simulink model "p1"  (R2020a)
settings: Solver=VariableStepAuto  StartTime=0.0  StopTime=10.0  RelTol=1e-3
settings Model: Creator=007  LastModifiedBy=007

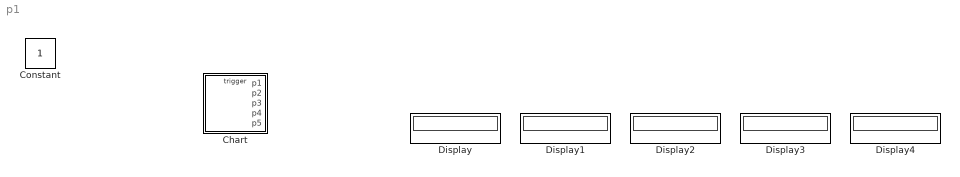
== system p1 ==
  Chart : Stateflow chart  TreatAsAtomicUnit=on
  Constant : Constant
  Display{,1..4} (5 alike) : Display

== stateflow chart p1/Chart ==
  state digit1
    state one
      entry:
      p1=1;
    state two
      entry:
      p1=2;
    state zero
      entry:
      p1=0;
    state three
      entry:
      p1=3;
    state four
      entry:
      p1=4;
    digit1.two -> digit1.three : inputclick
    digit1.zero -> digit1.one : inputclick
    digit1.one -> digit1.two : inputclick
    (default) -> digit1.zero
    digit1.four -> digit1.zero : inputclick/{digit2.inc2;}
    digit1.three -> digit1.four : inputclick
  state digit2
    state one
      entry:
      p2=1;
    state two
      entry:
      p2=2;
    state zero
      entry:
      p2=0;
    state three
      entry:
      p2=3;
    state four
      entry:
      p2=4;
    digit2.two -> digit2.three : inc2
    digit2.zero -> digit2.one : inc2
    digit2.one -> digit2.two : inc2
    (default) -> digit2.zero
    digit2.four -> digit2.zero : inc2/{digit3.inc3;}
    digit2.three -> digit2.four : inc2
  state digit3
    state one
      entry:
      p3=1;
    state two
      entry:
      p3=2;
    state zero
      entry:
      p3=0;
    state three
      entry:
      p3=3;
    state four
      entry:
      p3=4;
    digit3.two -> digit3.three : inc3
    digit3.zero -> digit3.one : inc3
    digit3.one -> digit3.two : inc3
    (default) -> digit3.zero
    digit3.four -> digit3.zero : inc3/{digit4.inc4;}
    digit3.three -> digit3.four : inc3
  state digit4
    state one
      entry:
      p4=1;
    state two
      entry:
      p4=2;
    state zero
      entry:
      p4=0;
    state three
      entry:
      p4=3;
    state four
      entry:
      p4=4;
    digit4.two -> digit4.three : inc4
    digit4.zero -> digit4.one : inc4
    digit4.one -> digit4.two : inc4
    (default) -> digit4.zero
    digit4.four -> digit4.zero : inc4/{digit5.inc5;}
    digit4.three -> digit4.four : inc4
  state digit5
    state one
      entry:
      p5=1;
    state two
      entry:
      p5=2;
    state zero
      entry:
      p5=0;
    state three
      entry:
      p5=3;
    state four
      entry:
      p5=4;
    digit5.two -> digit5.three : inc5
    digit5.zero -> digit5.one : inc5
    digit5.one -> digit5.two : inc5
    (default) -> digit5.zero
    digit5.four -> digit5.zero : inc5
    digit5.three -> digit5.four : inc5
  data: p1 output; p2 output; p3 output; p4 output; p5 output
  events: inputclick input RISING_EDGE_EVENT; inc2 local FUNCTION_CALL_EVENT; inc3 local FUNCTION_CALL_EVENT; inc4 local FUNCTION_CALL_EVENT; inc5 local FUNCTION_CALL_EVENT
